simulink model "gm_chorus"  (R2024a)
settings: Solver=VariableStepAuto  StartTime=0.0  StopTime=20  RelTol=1e-3
settings Model: Creator=fermata  LastModifiedBy=fermata
settings OptimizationCC: BlockReduction=off  ConditionallyExecuteInputs=off
settings DebuggingCC: InheritedTsInSrcMsg=none

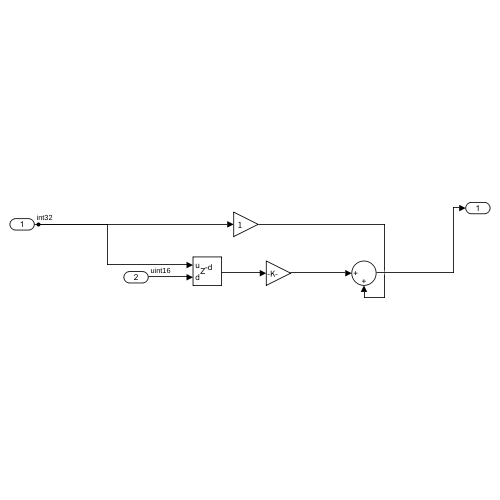
[thumbnail: Simulink's stored preview of the top-level diagram]
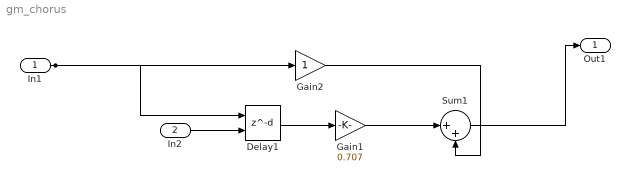
== system gm_chorus ==
  In1 : Inport  OutDataTypeStr=int32  PortDimensions=1  SampleTime=0.4
  In2 : Inport  Port=2  OutDataTypeStr=uint16  PortDimensions=1  SampleTime=0.4
  Delay1 : Delay  DelayLengthSource=Input port  DelayLength=1  DelayLengthUpperLimit=1024  InitialCondition=0
      settings: InputPortMap=u0,p1
  Gain1 : Gain  Gain=0.707  OutDataTypeStr=fixdt(1, 64, 31)
  Gain2 : Gain  OutDataTypeStr=fixdt(1, 64, 30)
  Sum1 : Sum  Inputs=|++  OutDataTypeStr=int32  RndMeth=Round  SaturateOnIntegerOverflow=on
  Out1 : Outport  SampleTime=0.4
  wires:
  In1/1 -> Gain2/1, Delay1/1
  In2/1 -> Delay1/2
  Delay1/1 -> Gain1/1
  Gain1/1 -> Sum1/1
  Gain2/1 -> Sum1/2
  Sum1/1 -> Out1/1
